simulink model "two_virtual_wheel_autocode"  (Simulink 7.8)
settings: Solver=FixedStepDiscrete  SolverMode=MultiTasking  StartTime=0.0  StopTime=tfinal  RelTol=1e-3
InitFcn:
  | two_virtual_wheel_params
undefined symbols (not defined in the file): b1, b2, DiscIntNeverNeededParam, Jw1, Jw2, k1, k2, SFunc_eTPU_quadraturedecoder_Script, SFunc_gpio_output_Script
libraries: rappid_ec_lib x2, simulink x2, rappid_lib x1
settings Model: Creator=Embed_Sys_course  LastModifiedBy=Embed_Sys_course  ExtModeTrigMode=oneshot  ExtModeArmWhenConnect=off
settings DataIOCC: LimitDataPoints=off  SignalLoggingName=sigsOut
settings OptimizationCC: BooleanDataType=off  InitFltsAndDblsToZero=on  OptimizeModelRefInitCode=on  LifeSpan=1
settings DebuggingCC: SaveWithParameterizedLinksMsg=none  SignalResolutionControl=TryResolveAllWithWarning  SolverPrmCheckMsg=none  MultiTaskDSMMsg=warning  MultiTaskCondExecSysMsg=none  FcnCallInpInsideContextMsg=Use local settings  StrictBusMsg=None
settings HardwareCC: TargetIntDivRoundTo=Zero  TargetEndianess=LittleEndian  TargetHWDeviceType=MATLAB Host  ProdEqTarget=off
settings RTWCC: SystemTargetFile=rappid.tlc  MakeCommand=rappid_make_rtw  TemplateMakefile=rappid_default_tmf  PostCodeGenCommand=rappid_analyzegencode(buildInfo)  Description=RAppID Toolbox MPC5554 Code Generation Target (rappid)  GenerateReport=on  ProcessScript=rappid_make_rtw_hook  IncludeHyperlinkInReport=on  LaunchReport=on  IncludeERTFirstTime=on  GenerateTraceInfo=on  GenerateTraceReport=on  GenerateTraceReportSl=on  GenerateTraceReportSf=on  GenerateTraceReportEml=on  GenerateCodeMetricsReport=on
settings CodeAppCC: IgnoreCustomStorageClasses=off
settings STFCustomTargetCC: ModelReferenceCompliant=off  GeneratePreprocessorConditionals=Use local settings  CombineOutputUpdateFcns=on  ERTCustomFileBanners=on  SupportContinuousTime=off  SupportNonInlinedSFcns=off  SystemTargetFile=rappid.tlc
settings ERTTargetCC: MultiwordLength=2048  ModelReferenceCompliant=off  ParMdlRefBuildCompliant=off  CompOptLevelCompliant=off  ConcurrentExecutionCompliant=off  ERTFirstTimeCompliant=off  ModelStepFunctionPrototypeControlCompliant=off  CPPClassGenCompliant=off  ExtModeMexFile=noextcomm  InlinedParameterPlacement=NonHierarchical  ERTCustomFileTemplate=example_file_process.tlc  ConvertIfToSwitch=off  SuppressUnreachableDefaultCases=off

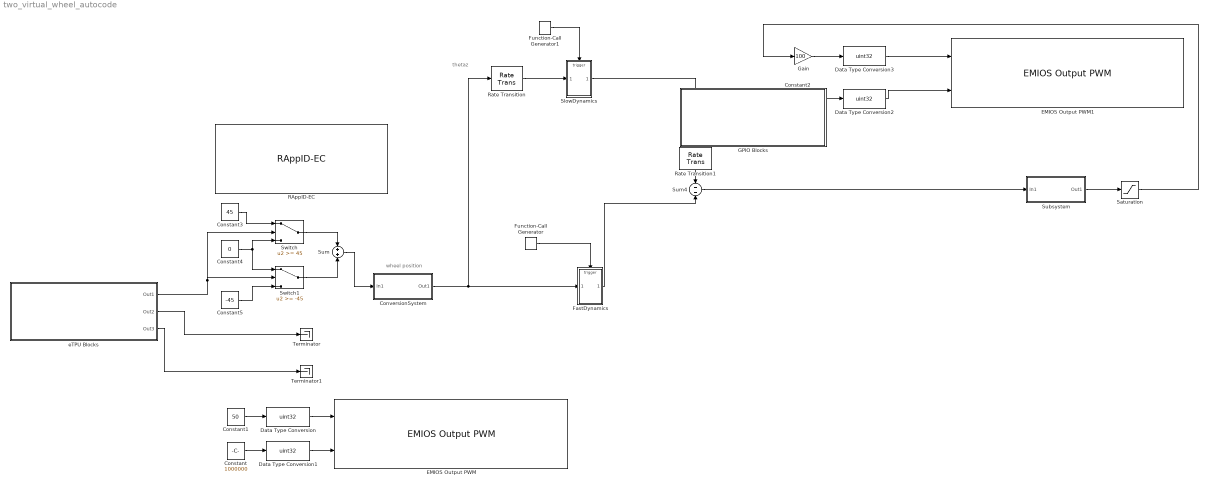
== system two_virtual_wheel_autocode ==
  note: wheel position
  note: thetaz
  Constant : Constant  Value=1000000  OutDataTypeStr=uint32
  Constant1 : Constant  Value=50  OutDataTypeStr=uint32
  Constant2 : Constant  Value=40000
  Constant3 : Constant  Value=45
  Constant4 : Constant  Value=0
  Constant5 : Constant  Value=-45
  ConversionSystem : Subsystem
  Data Type Conversion{,1..3} (4 alike) : DataTypeConversion  OutDataTypeStr=uint32
  EMIOS Output PWM : rappid_ec_lib/Peripheral Driver Blocks/eMIOS Blocks/EMIOS Output PWM  channelNo=12  emios_chan=12  A_init=50  B_init=1000000  clock=128  prescaler=1
  EMIOS Output PWM1 : rappid_ec_lib/Peripheral Driver Blocks/eMIOS Blocks/EMIOS Output PWM  channelNo=0  emios_chan=0  A_init=50  B_init=40000  clock=128  prescaler=1
  FastDynamics : Subsystem
  Function-Call Generator : simulink/Ports & Subsystems/Function-Call Generator  sample_time=0.002  numberOfIterations=1
  Function-Call Generator1 : simulink/Ports & Subsystems/Function-Call Generator  sample_time=0.02  numberOfIterations=1
  GPIO Blocks : Subsystem  AncestorBlock=rappid_ec_lib/Peripheral Driver Blocks/GPIO Blocks
      mask Display:
      | image(imread('freescale_logo.jpg'))
      | 
      | text(0.01,0.9,'GPIO')
  Gain : Gain  Gain=100
  RAppID-EC : rappid_lib/RAppID Initialization Blocks/RAppID-EC  Tag=RAppID  Priority=0  rtos=simpletarget  targetmcu=IntRAM  clockfrequency=128  basetaskpriority=20  systemcounter=0  systimer_isrpriority=1  systimer_period=0  isrstacksize=50  interruptdispatcher=None  stored_mdl_name=two_virtual_wheel_autocode
  Rate Transition : RateTransition
  Rate Transition1 : RateTransition
  Saturation : Saturate  UpperLimit=0.76  LowerLimit=0.24
  SlowDynamics : Subsystem
  Subsystem : Subsystem
  Sum : Sum
  Sum4 : Sum  Inputs=-|-  SaturateOnIntegerOverflow=on  InputSameDT=on  OutDataTypeStr=Inherit: Same as first input
  Switch : Switch  Threshold=45
  Switch1 : Switch  Threshold=-45
  Terminator : Terminator
  Terminator1 : Terminator
  eTPU Blocks : Subsystem  AncestorBlock=rappid_ec_lib/Peripheral Driver Blocks/eTPU Blocks
      mask Display:
      | image(imread('freescale_logo.jpg'))
      | 
      | text(0.01,0.9,'eTPU')
  wires:
  ConversionSystem/1(Out1) -> Rate Transition/1, FastDynamics/1(In1)
  Rate Transition1/1 -> Sum4/1
  Rate Transition/1 -> SlowDynamics/1(thetaz)
  SlowDynamics/1(torque1) -> Rate Transition1/1
  FastDynamics/1(torque2) -> Sum4/2
  Function-Call Generator1/1 -> SlowDynamics/Trigger
  Function-Call Generator/1 -> FastDynamics/Trigger
  Constant1/1 -> Data Type Conversion/1
  Data Type Conversion/1 -> EMIOS Output PWM/1
  Constant/1 -> Data Type Conversion1/1
  Data Type Conversion1/1 -> EMIOS Output PWM/2
  Subsystem/1(Out1) -> Saturation/1
  Saturation/1 -> Gain/1
  Constant2/1 -> Data Type Conversion2/1
  Data Type Conversion2/1 -> EMIOS Output PWM1/2
  Data Type Conversion3/1 -> EMIOS Output PWM1/1
  Gain/1 -> Data Type Conversion3/1
  Sum4/1 -> Subsystem/1(In1)
  eTPU Blocks/2(Out2) -> Terminator/1
  eTPU Blocks/3(Out3) -> Terminator1/1
  Constant3/1 -> Switch/1
  eTPU Blocks/1(Out1) -> Switch/2, Switch1/2
  Constant4/1 -> Switch/3, Switch1/1
  Constant5/1 -> Switch1/3
  Switch/1 -> Sum/1
  Switch1/1 -> Sum/2
  Sum/1 -> ConversionSystem/1(In1)

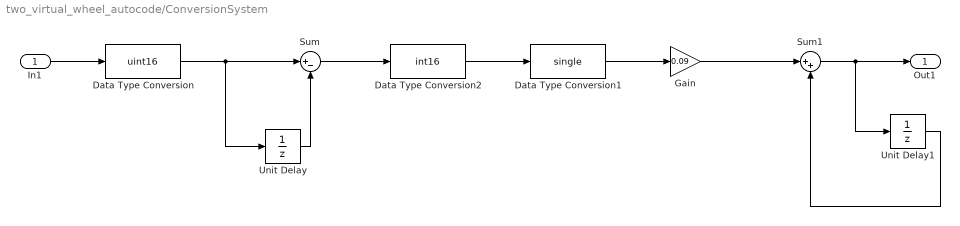
== system two_virtual_wheel_autocode/ConversionSystem ==
  In1 : Inport
  Data Type Conversion : DataTypeConversion  OutDataTypeStr=uint16
  Data Type Conversion1 : DataTypeConversion  OutDataTypeStr=single
  Data Type Conversion2 : DataTypeConversion  OutDataTypeStr=int16
  Gain : Gain  Gain=0.09
  Sum : Sum  Inputs=|+-
  Sum1 : Sum  Inputs=|++  AccumDataTypeStr=single  OutDataTypeStr=single
  Unit Delay : UnitDelay  SampleTime=-1
  Unit Delay1 : UnitDelay  SampleTime=-1
  Out1 : Outport
  wires:
  Unit Delay/1 -> Sum/2
  Sum/1 -> Data Type Conversion2/1
  Data Type Conversion2/1 -> Data Type Conversion1/1
  Data Type Conversion1/1 -> Gain/1
  Gain/1 -> Sum1/1
  Sum1/1 -> Out1/1, Unit Delay1/1
  Data Type Conversion/1 -> Sum/1, Unit Delay/1
  In1/1 -> Data Type Conversion/1
  Unit Delay1/1 -> Sum1/2

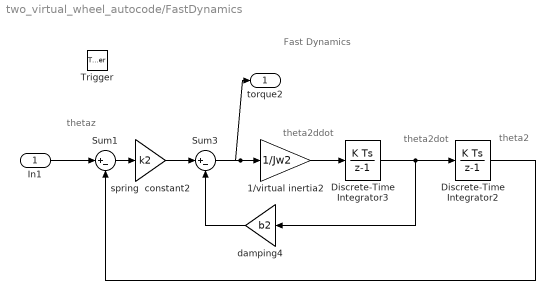
== system two_virtual_wheel_autocode/FastDynamics ==
  note: Fast Dynamics
  note: thetaz
  note: theta2ddot
  note: theta2dot
  note: theta2
  In1 : Inport
  Trigger : TriggerPort  TriggerType=function-call  PortDimensions=1
  1/virtual inertia2 : Gain  Gain=1/Jw2  SaturateOnIntegerOverflow=on  OutDataTypeStr=Inherit: Same as input  ParamDataTypeStr=Inherit: Same as input
  Discrete-Time Integrator2 : DiscreteIntegrator  SampleTime=-1  ICPrevOutput=DiscIntNeverNeededParam  ICPrevScaledInput=DiscIntNeverNeededParam
  Discrete-Time Integrator3 : DiscreteIntegrator  SampleTime=-1  ICPrevOutput=DiscIntNeverNeededParam  ICPrevScaledInput=DiscIntNeverNeededParam
  Sum1 : Sum  Inputs=|+-  SaturateOnIntegerOverflow=on  InputSameDT=on  OutDataTypeStr=Inherit: Same as first input
  Sum3 : Sum  Inputs=|+-  SaturateOnIntegerOverflow=on  InputSameDT=on  OutDataTypeStr=Inherit: Same as first input
  damping4 : Gain  Gain=b2  SaturateOnIntegerOverflow=on  OutDataTypeStr=Inherit: Same as input  ParamDataTypeStr=Inherit: Same as input
  spring  constant2 : Gain  Gain=k2  SaturateOnIntegerOverflow=on  OutDataTypeStr=Inherit: Same as input  ParamDataTypeStr=Inherit: Same as input
  torque2 : Outport
  wires:
  spring  constant2/1 -> Sum3/1
  damping4/1 -> Sum3/2
  Sum3/1 -> torque2/1, 1/virtual inertia2/1
  Discrete-Time Integrator3/1 -> Discrete-Time Integrator2/1, damping4/1
  1/virtual inertia2/1 -> Discrete-Time Integrator3/1
  Sum1/1 -> spring  constant2/1
  Discrete-Time Integrator2/1 -> Sum1/2
  In1/1 -> Sum1/1

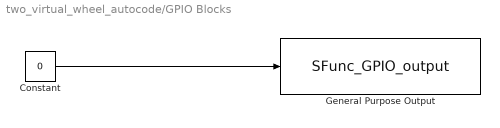
== system two_virtual_wheel_autocode/GPIO Blocks ==
  Constant : Constant  Value=0  OutDataTypeStr=boolean
  General Purpose Output : S-Function  InitFcn=SFunc_gpio_output_Script(bdroot(gcs)) ;  FunctionName=SFunc_GPIO_output  Parameters=char(gpoi_outputs),uint16(pinNum)  EnableBusSupport=off  mask(GPIO_Output){gpoi_outputs=205:   Primary Function "GPIO", pinNum=205}
      mask prompts: gpoi_outputs "Output Pin (GPO [ 0 - 213])"; pinNum "Pin Number"
      mask help: Select a General Purpose Output Pin as a Source (GPI [ 0 - 213]).
      mask init:
      | pinStr = get_param(gcb,'gpoi_outputs');
      | 
      | if strcmp(pinStr,'none')==0
      | 	pos =   findstr(pinStr,':');
      | 	pinVal = pinStr(1:pos(1)-1); 
      | 	set_param(gcb,'pinNum',pinVal);
      | 	st=['GPO [' pinVal, ']'];
      | else
      | 	set_param(gcb,'pinNum','');
      | 	st=['    No GPO Pin Selected'];
      | end
      mask Help: web([rappid_block_help,filesep,'gpio_output.htm']);
      mask StyleString: popup(93:   Primary Function "DSPI SCKA"|94:   Primary Function "DSPI SINA"|95:   Primary Function "DSPI SOUTA"|96:   Primary Function "DSPI PCSA0"|97:   Primary Function "DSPI PCSA1"|98:   Primary Function "DSPI PCSA2"|99:   Primary Function "DSPI PCSA3"|100:   Primary Function "DSPI PCSA4"|101:   Primary Function "DSPI PCSA5"|102:   Primary Function "DSPI SCKB"|103:   Primary Function "DSPI SINB"|104:   Primary Function "DSPI SOUTB"|105:   Primary Function "DSPI PCSB0"|106:   Primary Function "DSPI PCSB1"|107:   Primary Function "DSPI PCSB2"|108:   Primary Function "DSPI PCSB3"|109:   Primary Function "DSPI PCSB4"|110:   Primary Function "DSPI PCSB5"|114:   Primary Function "ETPUA CH0"|115:   Primary Function "ETPUA CH1"      |116:   Primary Function "ETPUA CH2"      |117:   Primary Function "ETPUA CH3"      |118:   Primary Function "ETPUA CH4"      |119:   Primary Function "ETPUA CH5"      |120:   Primary Function "ETPUA CH6"      |121:   Primary Function "ETPUA CH7"      |122:   Primary Function "ETPUA CH8"      |123:   Primary Function "ETPUA CH9"      |124:   Primary Function "ETPUA CH10"      |125:   Primary Function "ETPUA CH11"      |126:   Primary Function "ETPUA CH12"      |127:   Primary Function "ETPUA CH13"      |128:   Primary Function "ETPUA CH14" |129:   Primary Function "ETPUA CH15"|130:   Primary Function "ETPUA CH16"|131:   Primary Function "ETPUA CH17"|132:   Primary Function "ETPUA CH18"|133:   Primary Function "ETPUA CH19"|134:   Primary Function "ETPUA CH20"|135:   Primary Function "ETPUA CH21"|136:   Primary Function "ETPUA CH22"|137:   Primary Function "ETPUA CH23"|138:   Primary Function "ETPUA CH24"|139:   Primary Function "ETPUA CH25"|140:   Primary Function "ETPUA CH26"|141:   Primary Function "ETPUA CH27"|142:   Primary Function "ETPUA CH28"|143:   Primary Function "ETPUA CH29"|144:   Primary Function "ETPUA CH30"|145:   Primary Function "ETPUA CH31"|147:   Primary Function "ETPUB CH0"|148:   Primary Function "ETPUB CH1"|149:   Primary Function "ETPUB CH2"|150:   Primary Function "ETPUB CH3"|151:   Primary Function "ETPUB CH4"|152:   Primary Function "ETPUB CH5"|153:   Primary Function "ETPUB CH6"|154:   Primary Function "ETPUB CH7"|155:   Primary Function "ETPUB CH8"|156:   Primary Function "ETPUB CH9"|157:   Primary Function "ETPUB CH10"|158:   Primary Function "ETPUB CH11"|159:   Primary Function "ETPUB CH12"|160:   Primary Function "ETPUB CH13"|161:   Primary Function "ETPUB CH14"|162:   Primary Function "ETPUB CH15"|163:   Primary Function "ETPUB CH16"|164:   Primary Function "ETPUB CH17"|165:   Primary Function "ETPUB CH18"|166:   Primary Function "ETPUB CH19"|167:   Primary Function "ETPUB CH20"|168:   Primary Function "ETPUB CH21"|169:   Primary Function "ETPUB CH22"|170:   Primary Function "ETPUB CH23"|171:   Primary Function "ETPUB CH24"|172:   Primary Function "ETPUB CH25"|173:   Primary Function "ETPUB CH26"|174:   Primary Function "ETPUB CH27"|175:   Primary Function "ETPUB CH28"|176:   Primary Function "ETPUB CH29"|177:   Primary Function "ETPUB CH30"|178:   Primary Function "ETPUB CH31"|179:   Primary Function "EMIOS CH0"|180:   Primary Function "EMIOS CH1"|181:   Primary Function "EMIOS CH2"|182:   Primary Function "EMIOS CH3"|183:   Primary Function "EMIOS CH4"|184:   Primary Function "EMIOS CH5"|185:   Primary Function "EMIOS CH6"|186:   Primary Function "EMIOS CH7"|187:   Primary Function "EMIOS CH8"|188:   Primary Function "EMIOS CH9"|189:   Primary Function "EMIOS CH10"|190:   Primary Function "EMIOS CH11"|191:   Primary Function "EMIOS CH12"|192:   Primary Function "EMIOS CH13"|193:   Primary Function "EMIOS CH14"|194:   Primary Function "EMIOS CH15"|195:   Primary Function "EMIOS CH16"|196:   Primary Function "EMIOS CH17"|197:   Primary Function "EMIOS CH18"|198:   Primary Function "EMIOS CH19"|199:   Primary Function "EMIOS CH20"|200:   Primary Function "EMIOS CH21"|201:   Primary Function "EMIOS CH22"|202:   Primary Function "EMIOS CH23"|203:   Primary Function "GPIO"|204:   Primary Function "GPIO"|205:   Primary Function "GPIO"|206:   Primary Function "GPIO"|207:   Primary Function "GPIO"|none),edit
      mask Display:
      | disp(st);
      | port_label('input',1,'output')
  wires:
  Constant/1 -> General Purpose Output/1

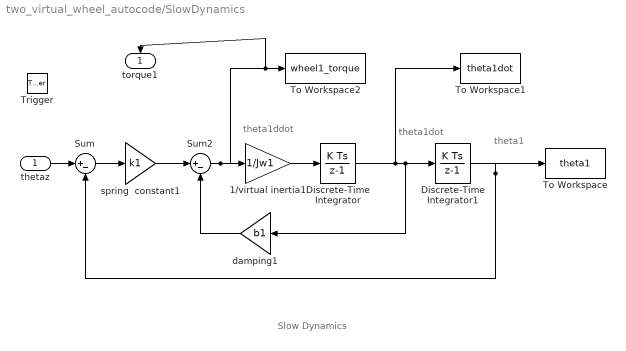
== system two_virtual_wheel_autocode/SlowDynamics ==
  note: Slow Dynamics
  note: theta1ddot
  note: theta1dot
  note: theta1
  thetaz : Inport
  Trigger : TriggerPort  TriggerType=function-call  PortDimensions=1
  1/virtual inertia1 : Gain  Gain=1/Jw1  SaturateOnIntegerOverflow=on  OutDataTypeStr=Inherit: Same as input  ParamDataTypeStr=Inherit: Same as input
  Discrete-Time Integrator : DiscreteIntegrator  SampleTime=-1  ICPrevOutput=DiscIntNeverNeededParam  ICPrevScaledInput=DiscIntNeverNeededParam
  Discrete-Time Integrator1 : DiscreteIntegrator  SampleTime=-1  ICPrevOutput=DiscIntNeverNeededParam  ICPrevScaledInput=DiscIntNeverNeededParam
  Sum : Sum  Inputs=|+-  SaturateOnIntegerOverflow=on  InputSameDT=on  OutDataTypeStr=Inherit: Same as first input
  Sum2 : Sum  Inputs=|+-  SaturateOnIntegerOverflow=on  InputSameDT=on  OutDataTypeStr=Inherit: Same as first input
  To Workspace : ToWorkspace  VariableName=theta1  SampleTime=-1  SaveFormat=Structure With Time
  To Workspace1 : ToWorkspace  VariableName=theta1dot  SampleTime=-1  SaveFormat=Structure With Time
  To Workspace2 : ToWorkspace  VariableName=wheel1_torque  SampleTime=-1  SaveFormat=Structure With Time
  damping1 : Gain  Gain=b1  SaturateOnIntegerOverflow=on  OutDataTypeStr=Inherit: Same as input  ParamDataTypeStr=Inherit: Same as input
  spring  constant1 : Gain  Gain=k1  SaturateOnIntegerOverflow=on  OutDataTypeStr=Inherit: Same as input  ParamDataTypeStr=Inherit: Same as input
  torque1 : Outport
  wires:
  damping1/1 -> Sum2/2
  Sum2/1 -> 1/virtual inertia1/1, To Workspace2/1, torque1/1
  spring  constant1/1 -> Sum2/1
  Discrete-Time Integrator/1 -> Discrete-Time Integrator1/1, damping1/1, To Workspace1/1
  1/virtual inertia1/1 -> Discrete-Time Integrator/1
  Sum/1 -> spring  constant1/1
  Discrete-Time Integrator1/1 -> Sum/2, To Workspace/1
  thetaz/1 -> Sum/1

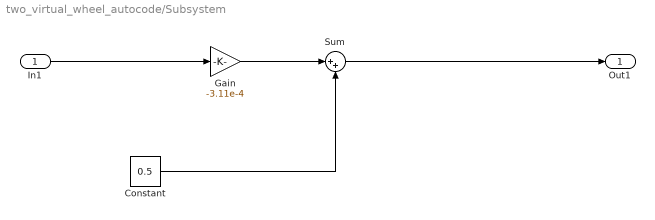
== system two_virtual_wheel_autocode/Subsystem ==
  In1 : Inport
  Constant : Constant  Value=0.5
  Gain : Gain  Gain=-3.11e-4
  Sum : Sum  Inputs=|++
  Out1 : Outport
  wires:
  Gain/1 -> Sum/1
  Constant/1 -> Sum/2
  In1/1 -> Gain/1
  Sum/1 -> Out1/1

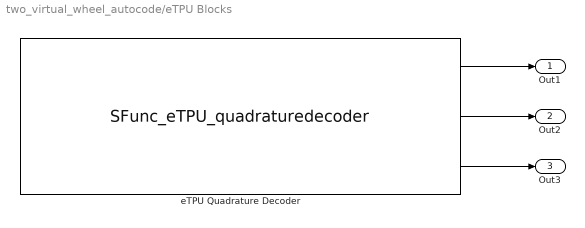
== system two_virtual_wheel_autocode/eTPU Blocks ==
  eTPU Quadrature Decoder : S-Function  Priority=-100000000  InitFcn=SFunc_eTPU_quadraturedecoder_Script;  FunctionName=SFunc_eTPU_quadraturedecoder  Parameters=uint8(etpu) ,uint8(chan),uint32(speed_max_rpm),uint32(pcincrements_per_rev),uint8(pcscaling)  EnableBusSupport=off  mask(SFunc_eTPU_quadraturedecoder){etpu=0, chan=3, speed_max_rpm=1000, pcincrements_per_rev=4000, pcscaling=4}
      mask prompts: chan "Channel"; speed_max_rpm "Max Speed (rpm)"; pcincrements_per_rev "Position Counter Increments per Revolution (4 X lines on motor)"; pcscaling "Position Count Scaling"
      mask help: Implements the quadrature decoder functionality based on phase A and phase B encoder signals typicaly used for controlling DC motors. Outputs Position Counts (24-bit counter which rolls over on overflow), Angular Velocity in rpm and Direction of motor at every time-step. Right-click on the block and see block help for usage details
      mask init:
      | etpudm = ['eTPU: ' get_param(gcb,'etpu')];
      | chandm = ['Channel: ' num2str(str2num(get_param(gcb,'chan')) + (str2num(get_param(gcb,'etpu'))*64))];
      | secchandm = ['Secondary Channel: ' num2str(str2num(get_param(gcb,'chan')) + (str2num(get_param(gcb,'etpu'))*64)+1)];
      | speed_max_rpmdm = ['Max Speed (rpm): ' num2str(get_value(get_param(gcb,'speed_max_rpm')))];
      | pcincrements_per_revdm = ['Position Counter Increments per Revolution (4 X lines on motor): ' num2str(get_value(get_param(gcb,'pcincrements_per_rev')))];
      | pcscalingdm = ['Position Counts Scaling): PositionCounts X ' get_param(gcb,'pcscaling')];
      | rp_set_cur_model(bdroot(gcb));
      mask Help: web([rappid_block_help,filesep,'SFunc_eTPU_quadraturedecoder.htm']);
      mask StyleString: popup(0|1),popup(0|1|2|3|4|5|6|7|8|9|10|11|12|13|14|15|16|17|18|19|20|21|22|23|24|25|26|27|28|29|30|31),edit,edit,popup(1|2|3|4|5|6|7|8|9|10|11|12|13|14|15|16)
      mask Display:
      | disp(['eTPU Quadrature Decoder \n  Set3 functions DC Motor Controls \n\n'  etpudm '\n' chandm '\n' secchandm '\n' speed_max_rpmdm '\n' pcincrements_per_revdm '\n' pcscalingdm '\n' 'FUNCTION NUMBER: FS_ETPU_QD_FUNCTION_NUMBER' '\n' 'ENTRY TABLE ENCODING: FS_ETPU_QD_TABLE_SELECT' '\n']);
      | 
      | 
      | port_label('output',1,'Position Count');
      | port_label('output',2,'Angular Velocity (rpm)');
      | port_label('output',3,'Direction (0-pos: 1-neg)');
  Out1 : Outport
  Out2 : Outport  Port=2
  Out3 : Outport  Port=3
  wires:
  eTPU Quadrature Decoder/1 -> Out1/1
  eTPU Quadrature Decoder/2 -> Out2/1
  eTPU Quadrature Decoder/3 -> Out3/1
